simulink model "EffectuatorIntegratedWithDemonstrator"  (R2020a)
settings: Solver=FixedStepDiscrete  StartTime=0.0  StopTime=inf  FixedStep=Ts  RelTol=1e-3
InitFcn:
  | %% Verwende vordefinierte Setpoints (Kreis mit Z-Komponente)
  | 
  | % Config
  | numCircles = 3;
  | scale=6;
  | %Versuch symmetrische Setpunkte zu setzen
  | pointsPerCircle =scale*(4+3*numCircles)+2;
  | 
  | r = 50;
  | m_x = r;
  | m_y = r;
  | 
  | % //
  | s = linspace(0,2*pi,pointsPerCircle);
  | 
  | setPoints_x = [];
  | setPoints_y = [];
  | 
  | for ii=1:numCircles
  | 
  | setPoints_x = [setPoints_x (-cos(s(1:floor(pointsPerCircle / 2))).*r + m_x + 2*r*(ii-1))]; %#ok<AGROW>
  | setPoints_y = [setPoints_y (sin(s).*r+m_y)]; %#ok<AGROW>pointsPerCircle / 2
  | 
  | end
  | 
  | setPoints_x = [setPoints_x flip(setPoints_x(1:end))];
  | 
  | % Loeschen doppelter y-Werte (Kreisuebergang)
  | setPoints_x(pointsPerCircle .* [1:numCircles]) = [];
  | setPoints_y(pointsPerCircle .* [1:numCircles]) = [];
  | 
  | % setPoints_x= [linspace(0,setPoints_x(19),19) setPoints_x(20:end)];
  | % setPoints_y= [linspace(0,setPoints_y(19),19) setPoints_y(20:end)];
  | 
  | % Array Elemente verschieben
  | % setPoints_x = circshift(setPoints_x,-pointsPerCircle/4,2);
  | % setPoints_y = circshift(setPoints_y,-pointsPerCircle/4,2);
  | 
  | z = zeros(1,size(setPoints_x,2));
  | z_x = -5:5;
  | z_y = -z_x.^2 + 25;
  | z_idx = 90;
  | z_idx2 = 210;
  | z(z_idx:z_idx+length(z_x)-1) = z_y;
  | z(z_idx2:z_idx2+length(z_x)-1) = z_y;
  | % z = [z_y z];
  | setPoints_z = z;
  | 
  | % setPoints_x = [zeros(1,length(z_y)) setPoints_x];
  | % setPoints_y = [setPoints_y(1,1)*ones(1,length(z_y)) setPoints_y];
  | 
  | % Umrechnung der Einheiten für Demonstrator
  | % setPoints_x = setPoints_x ./ 1000;
  | % setPoints_y = setPoints_y ./ 1000;
  | % setPoints_z = setPoints_z ./ 1000;
  | 
  | 
  | %{
  | plot(setPoints_x,setPoints_y);
  | fig = figure;
  | plot3(setPoints_x(1:end-1),setPoints_y(1:end-1),setPoints_z(1:end-1));
  | 
  | ax = gca;
  | ax.YDir = 'reverse';
  | ax.ZDir = 'reverse';
  | %}
  | 
  | % setPoints_z = zeros(1,size(setPoints_x,2));
  | 
  | setP_mat = [setPoints_x;setPoints_y;setPoints_z];
  | %Dauerlauftest zehn Durchgänge
  | %setP_mat = repmat(setP_mat, 1, 10);
  | setP_mat = setP_mat(:,2:end);
StartFcn:
  | close all;
model workspace (MAT data in the model file):
  MvmtPerfEval_collectVal = Simulink.Parameter
  MvmtPerfEval_collectVal.Value = 0.65
  MvmtPerfEval_collectVal.Description = '- Anteil eines Interpolationssegments (0,1)
    | - Nach Abarbeitung des spezifizierten Anteils wird gemeinsame Performance aller Agenten
    | vom Dispatcher geladen
    | 
    | - (!!!) Wert MUSS größer sein als MvmtPerfEval_sendOwnVal'
  MvmtPerfEval_collectVal.DataType = 'auto'
  MvmtPerfEval_collectVal.Min = 0
  MvmtPerfEval_collectVal.Max = 1
  MvmtPerfEval_collectVal.Dimensions = [1 1]
  MvmtPerfEval_sendOwnVal = Simulink.Parameter
  MvmtPerfEval_sendOwnVal.Value = 0.6
  MvmtPerfEval_sendOwnVal.Description = '- Anteil eines Interpolationssegments (0,1)
    | - Nach Abarbeitung des spezifizierten Anteils wird Perfomance Kennzahl an Dispatcher übermittelt
    | 
    | - (!!!) Wert MUSS kleiner sein als MvmtPerfEval_collectVal'
  MvmtPerfEval_sendOwnVal.DataType = 'auto'
  MvmtPerfEval_sendOwnVal.Min = 0
  MvmtPerfEval_sendOwnVal.Max = 1
  MvmtPerfEval_sendOwnVal.Dimensions = [1 1]
  PerfEval_numTicks_enable = Simulink.Parameter
  PerfEval_numTicks_enable.Value = 10
  PerfEval_numTicks_enable.Description = 'Anzahl der Ticks (Integrationsschritte), bevor die Performance ausgewertet wird
    | (unabhängig vom Senden des Werts an den Dispatcher)'
  PerfEval_numTicks_enable.DataType = 'auto'
  PerfEval_numTicks_enable.Dimensions = [1 1]
  Segmentregler_I_Gain = Simulink.Parameter
  Segmentregler_I_Gain.Value = 1
  Segmentregler_I_Gain.DataType = 'auto'
  Segmentregler_I_Gain.Dimensions = [1 1]
  Segmentregler_P_Gain = Simulink.Parameter
  Segmentregler_P_Gain.Value = 0
  Segmentregler_P_Gain.DataType = 'auto'
  Segmentregler_P_Gain.Dimensions = [1 1]
  Segmentregler_minVel_enable = Simulink.Parameter
  Segmentregler_minVel_enable.Value = 0.1
  Segmentregler_minVel_enable.DataType = 'auto'
  Segmentregler_minVel_enable.Dimensions = [1 1]
  Segmentregler_numTicks_enable = Simulink.Parameter
  Segmentregler_numTicks_enable.Value = 30
  Segmentregler_numTicks_enable.Description = 'Anzahl der Ticks (Integrationsschritte), bevor der Segmentregler aktiv wird'
  Segmentregler_numTicks_enable.DataType = 'auto'
  Segmentregler_numTicks_enable.Dimensions = [1 1]
  Ts = Simulink.Parameter
  Ts.Value = 0.005
  Ts.Description = 'Sampling Time'
  Ts.DataType = 'auto'
  Ts.Dimensions = [1 1]
  maxPos_x = Simulink.Parameter
  maxPos_x.Value = 300
  maxPos_x.Description = 'Grenze des Arbeitsbereichs (maximaler Wert der Koordinate)'
  maxPos_x.DataType = 'auto'
  maxPos_x.Dimensions = [1 1]
  maxPos_y = Simulink.Parameter
  maxPos_y.Value = 150
  maxPos_y.Description = 'Grenze des Arbeitsbereichs (maximaler Wert der Koordinate)'
  maxPos_y.DataType = 'auto'
  maxPos_y.Dimensions = [1 1]
  maxPos_z = Simulink.Parameter
  maxPos_z.Value = 50
  maxPos_z.Description = 'Grenze des Arbeitsbereichs (maximaler Wert der Koordinate)'
  maxPos_z.DataType = 'auto'
  maxPos_z.Dimensions = [1 1]
  maxVectorLengths = Simulink.Parameter
  maxVectorLengths.Value = 16376
  maxVectorLengths.DataType = 'auto'
  maxVectorLengths.Dimensions = [1 1]
  minAllowedVelSaturation = Simulink.Parameter
  minAllowedVelSaturation.Value = 0.05
  minAllowedVelSaturation.Description = 'Minimaler Saturation-Wert für den Geschwindigkeits-PID-Regler
    | (auch bei Sollgeschwindigkeit soll Fehlerkorrektur möglich sein)'
  minAllowedVelSaturation.DataType = 'auto'
  minAllowedVelSaturation.Dimensions = [1 1]
  numAxes = Simulink.Parameter
  numAxes.Value = 4
  numAxes.DataType = 'auto'
  numAxes.Dimensions = [1 1]
undefined symbols (not defined in the file or in its folder): DiscIntNeverNeededParam, VelOverride
libraries: simulink x20, vrlib x5, sldrtlib x2, xpcrtudplib x2, dspnetwork x2, ptplib x1, etargetslib x1, xpcutilitieslib x1
(part 1 of 5)
settings Model: xpc_rtwmakecfg_data=_xpcnblib__xpcetherlib__xpcether8255xlib__xpcetherGbElib__xpciplib_  EnablePacing=on  PacingRate=10  Creator=Daniel  LastModifiedBy=Hiwi
settings DataIOCC: ReturnWorkspaceOutputs=off
settings DebuggingCC: AlgebraicLoopMsg=none  ArithmeticOperatorsInVariantConditions=warning
settings SFSimCC: CustomCodeUndefinedFunction=UseInterfaceOnly

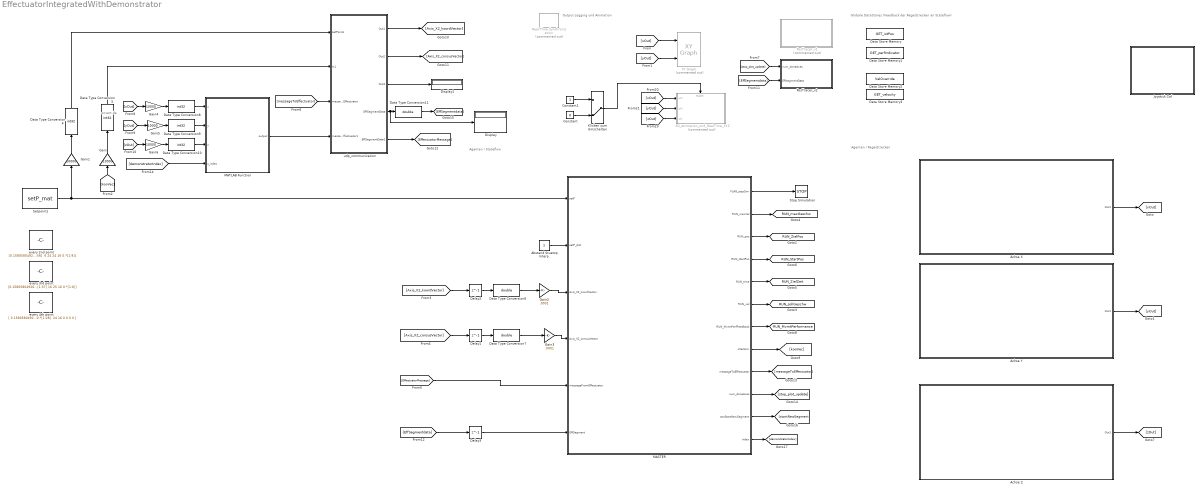
== system EffectuatorIntegratedWithDemonstrator ==
  note: onvert da
  note: Globale DataStores (Feedback der Regelstrecken an Stateflow)
  note: Agenten / Regelstrecken
  note: Agenten / Stateflow
  note: Output-Logging und Animation
  3D_Animation_und_RealTime_XYZ : Subsystem  Commented=on
  Abstand Stuetzp. Interp. : Constant
  Achse X : Subsystem
  Achse Y : Subsystem
  Achse Z : Subsystem
  Constant : Constant  Value=0
  Constant1 : Constant
  Data Store Memory : DataStoreMemory  DataStoreName=GET_istPos  ReadBeforeWriteMsg=warning  WriteAfterWriteMsg=warning  WriteAfterReadMsg=warning  InitialValue=zeros(1,numAxes)  ShowAdditionalParam=off  OutDataTypeStr=double
  Data Store Memory1 : DataStoreMemory  DataStoreName=GET_perfIndicator  ReadBeforeWriteMsg=warning  WriteAfterWriteMsg=warning  WriteAfterReadMsg=warning  InitialValue=zeros(1,numAxes)  ShowAdditionalParam=off  OutDataTypeStr=double
  Data Store Memory2 : DataStoreMemory  DataStoreName=VelOverride  ReadBeforeWriteMsg=warning  WriteAfterWriteMsg=warning  WriteAfterReadMsg=warning  InitialValue=ones(1,numAxes)  ShowAdditionalParam=off  OutDataTypeStr=double
  Data Store Memory3 : DataStoreMemory  DataStoreName=GET_velocity  ReadBeforeWriteMsg=warning  WriteAfterWriteMsg=warning  WriteAfterReadMsg=warning  InitialValue=zeros(1,numAxes)  ShowAdditionalParam=off  OutDataTypeStr=double
  Data Type Conversion{4..5,8..10} (5 alike) : DataTypeConversion  OutDataTypeStr=int32
  Data Type Conversion11 : DataTypeConversion  OutDataTypeStr=double
  Data Type Conversion6 : DataTypeConversion  OutDataTypeStr=double
  Data Type Conversion7 : DataTypeConversion  OutDataTypeStr=double
  Delay1 : Delay  DelayLength=1
  Delay2 : Delay  DelayLength=1
  Delay3 : Delay  DelayLength=1
  Display : Display
  Display1 : Display
  Gain{,1,4..6} (5 alike) : Gain  Gain=10000
  Gain2 : Gain  Gain=.0001
  Gain3 : Gain  Gain=.0001
  Joystick Ctrl : Subsystem
  Klicken zum Umschalten : ManualSwitch  CurrentSetting=0
  MASTER : Stateflow chart  TreatAsAtomicUnit=on
  MATLAB Function : MATLAB Function  TreatAsAtomicUnit=on
  PosTracer_v1 : Stateflow chart  Commented=on  TreatAsAtomicUnit=on
  PosTracer_v2 : Stateflow chart  TreatAsAtomicUnit=on
  Real-Time Synchronization : sldrtlib/Real-Time Synchronization  Commented=on  SampleTime=0.005  MaxMissedTicks=1000  ShowMissedTicks=off  YieldWhenWaiting=off
  Setpoints : Constant  Value=setP_mat
  Stop Simulation : Stop
  XY Graph : simulink/Sinks/XY Graph  Commented=on  xmin=0  xmax=maxPos_x  ymin=0  ymax=maxPos_y  st=-1
  every 2nd point : Constant  Value="[0.158058049265208 1.41653299797949 3.90170726358966 7.55083189543181 12.2717689920885 17.9453181203890 24.4282260448289 31.5568037737996 39.1510595946841 47.0192437415090 54.9626899454031 62.7808316220237 70.2762660406497 77.2597386081334 83.5549214179519 89.0028654092606 93.4660137219791 96.8316749134364 99.0148683402318 99.9604698613651 100.158058049265 101.416532997979 103.901707263590 107.550831895432 112.271768992089 117.945318120389 124.428226044829  131.556803773800 139.151059594684 147.019243741509 154.962689945403 162.780831622024 170.276266040650 177.259738608133 183.554921417952 189.002865409261 193.466013721979 196.831674913436 199.014868340232 200 200.631232903183 202.508993413611  205.585869362543 209.784171736462 214.997896271529 221.095399988758 227.922725089204 235.307486283104 243.063223400547  250.994109383254 258.899894783877 266.580963927603 273.843375071425  280.503757300526 286.393940518475 291.365201627153 295.292019683276 298.075245216371 299.644603685099 299.960469861365  299.014868340232 296.831674913436  293.466013721979 289.002865409261 283.554921417952 277.259738608133 270.276266040650 262.780831622024 254.962689945403 247.019243741509 239.151059594684 231.556803773800 224.428226044829 217.945318120389 212.271768992088 207.550831895432 203.901707263590 201.416532997980 200.158058049265 199.644603685099 198.075245216371 195.292019683276 191.365201627153 186.393940518475 180.503757300526 173.843375071425 166.580963927603 158.899894783878 150.994109383254 143.063223400547 135.307486283104 127.922725089204 121.095399988758 114.997896271529 109.784171736462 105.585869362543 102.508993413611 100.631232903183 100 99.6446036850987 98.0752452163710 95.2920196832762 91.3652016271529 86.3939405184747 80.5037573005262 73.8433750714253 66.5809639276034 58.8998947838775 50.9941093832535 43.0632234005466 35.3074862831040 27.9227250892044 21.0953999887576 14.9978962715287 9.78417173646176 5.58586936254341 2.50899341361087 0.631232903183332 ; 53.9725083485857 61.8172219266452 69.3635587325321 76.4209789226310 82.8112874635188 88.3731334346954 92.9660840289831 96.4741703848694 98.8088157209525 99.9110718390967 99.7531075261214  98.3389112729019 95.7041905677017 91.9154703065138 87.0684130849309 81.2854037830280 74.7124594308362 67.5155423781912 59.8763698588976 51.9878257548463 44.0490904099048 36.2606114624487 28.8190426795736 21.9122785839615 15.7147102456794 10.3828220269213  6.05124045887832 2.82933501389326 0.798456601078975 0.00988351149672440 0.483526676374908 2.20742692971196 5.13805696903938 9.20142039004195 14.2949200451625 20.2899485514145 27.0351355388511 34.3601696488886 42.0800987796393 50 57.9199012203608 65.6398303511114 72.9648644611489 79.7100514485855 85.7050799548375 90.7985796099580 94.8619430309606 97.7925730702880 99.5164733236251 99.9901164885033 99.2015433989211 97.1706649861067 93.9487595411217 89.6171779730787 84.2852897543207 78.0877214160385 71.1809573204264 63.7393885375513 55.9509095900952 48.0121742451537 40.1236301411024 32.4844576218088 25.2875405691639 18.7145962169720 12.9315869150691 8.08452969348616 4.29580943229828 1.66108872709815 0.246892473878624 0.0889281609033432 1.19118427904746 3.52582961513065 7.03391597101695 11.6268665653046 17.1887125364812 23.5790210773690 30.6364412674680 38.1827780733548 46.0274916514143 53.9725083485857 61.8172219266452 69.3635587325321 76.4209789226310 82.8112874635188 88.3731334346954 92.9660840289831 96.4741703848694 98.8088157209525 99.9110718390967 99.7531075261214 98.3389112729019 95.7041905677017  91.9154703065138 87.0684130849309 81.2854037830280 74.7124594308362 67.5155423781912 59.8763698588976 51.9878257548463 44.0490904099048 36.2606114624487 28.8190426795736 21.9122785839615 15.7147102456794 10.3828220269213 6.05124045887832 2.82933501389326 0.798456601078975 0.00988351149672440 0.483526676374908 2.20742692971196 5.13805696903938 9.20142039004195 14.2949200451625 20.2899485514145 27.0351355388511 34.3601696488886 42.0800987796393 ; 0.*[1:45] 16 24 24 16 0.*[1:56]  6 24 24 16 0.*[1:9]]"  VectorParams1D=off
  every 3rd point : Constant  Value="[0.158058049265208 2.50899341361087 7.55083189543181  14.9978962715287 24.4282260448289 35.3074862831040 47.0192437415090 58.8998947838775 70.2762660406497 80.5037573005262 89.0028654092606 95.2920196832762 99.0148683402318 100 101.416532997979 105.585869362543 112.271768992089 121.095399988758 131.556803773800 143.063223400547 154.962689945403 166.580963927603 177.259738608133 186.393940518475 193.466013721979 198.075245216371 200 201.416532997980 205.585869362543 212.271768992088 221.095399988758 231.556803773800 243.063223400547 254.962689945403 266.580963927603 277.259738608133 286.393940518475 293.466013721979 298.075245216371 299.960469861365 299.014868340232 295.292019683276 289.002865409261 280.503757300526 270.276266040650 258.899894783877 247.019243741509 235.307486283104 224.428226044829 214.997896271529 207.550831895432 202.508993413611 200.158058049265 199.014868340232 195.292019683276 189.002865409261 180.503757300526 170.276266040650 158.899894783878 147.019243741509 135.307486283104 124.428226044829 114.997896271529 107.550831895432 102.508993413611 100.158058049265 99.6446036850987 96.8316749134364 91.3652016271529 83.5549214179519 73.8433750714253 62.7808316220237 50.9941093832535 39.1510595946841 27.9227250892044 17.9453181203890 9.78417173646176 3.90170726358966 0.631232903183332; 53.9725083485857 65.6398303511114 76.4209789226310 85.7050799548375 92.9660840289831 97.7925730702880 99.9110718390967 99.2015433989211 95.7041905677017 89.6171779730787 81.2854037830280 71.1809573204264 59.8763698588976 48.0121742451537 36.2606114624487 25.2875405691639 15.7147102456794 8.08452969348616 2.82933501389326 0.246892473878624 0.483526676374908 3.52582961513065 9.20142039004195 17.1887125364812 27.0351355388511 38.1827780733548 50 61.8172219266452 72.9648644611489 82.81128746351 88 90.7985796099580 96.4741703848694 99.5164733236251 99.7531075261214 97.1706649861067 91.9154703065138 84.2852897543207 74.7124594308362 63.7393885375513 51.9878257548463 40.1236301411024 28.8190426795736 18.7145962169720 10.3828220269213 4.29580943229828 0.798456601078975 0.0889281609033432 2.20742692971196 7.03391597101695 14.2949200451625 23.5790210773690 34.3601696488886 46.0274916514143 57.9199012203608 69.3635587325321 79.7100514485855 88.3731334346954 94.8619430309606 98.8088157209525 99.9901164885033 98.3389112729019 93.9487595411217 87.0684130849309 78.0877214160385 67.5155423781912 55.9509095900952 44.0490904099048 32.4844576218088  21.9122785839615 12.9315869150691 6.05124045887832 1.66108872709815 0.00988351149672440 1.19118427904746 5.13805696903938 11.6268665653046 30.6364412674680 42.0800987796393;0.*[1:30] 16 25 16 0.*[1:37] 16 25 16 0.*[1:6]]"  VectorParams1D=off
  every 4th point : Constant  Value="[ 0.158058049265208 3.90170726358966 12.2717689920885 24.4282260448289 39.1510595946841 54.9626899454031 70.2762660406497 83.5549214179519  93.4660137219791 99.0148683402318 100.158058049265  103.901707263590 112.271768992089 124.428226044829 139.151059594684 154.962689945403  170.276266040650 183.554921417952 193.466013721979 199.014868340232 200.631232903183  205.585869362543 214.997896271529 227.922725089204 243.063223400547 258.899894783877 273.843375071425 286.393940518475 295.292019683276 299.644603685099 299.014868340232 293.466013721979 283.554921417952 270.276266040650 254.962689945403 239.151059594684 224.428226044829 212.271768992088 203.901707263590 200.158058049265 198.075245216371 191.365201627153 180.503757300526 166.580963927603 150.994109383254 135.307486283104 121.095399988758 109.784171736462 102.508993413611 100 98.0752452163710 91.3652016271529 80.5037573005262 66.5809639276034 50.9941093832535 35.3074862831040 21.0953999887576 9.78417173646176 2.50899341361087; 53.9725083485857 69.3635587325321 82.8112874635188 92.9660840289831 98.8088157209525 99.7531075261214 95.7041905677017 87.0684130849309 74.7124594308362 59.8763698588976 44.0490904099048 28.8190426795736 15.7147102456794 6.05124045887832 0.798456601078975 0.483526676374908 5.13805696903938 14.2949200451625 27.0351355388511  42.0800987796393 57.9199012203608 72.9648644611489  85.7050799548375 94.8619430309606 99.5164733236251 99.2015433989211  93.9487595411217 84.2852897543207 71.1809573204264 55.9509095900952 40.1236301411024 25.2875405691639 12.9315869150691  4.29580943229828 0.246892473878624  1.19118427904746 7.03391597101695 17.1887125364812 30.6364412674680 46.0274916514143 61.8172219266452 76.4209789226310 88.3731334346954 96.4741703848694 99.9110718390967 98.3389112729019 91.9154703065138  81.2854037830280 67.5155423781912 51.9878257548463 36.2606114624487 21.9122785839615 10.3828220269213 2.82933501389326 0.00988351149672440 2.20742692971196 9.20142039004195 20.2899485514145 34.3601696488886;0.*[1:23] 24 16 0.*[1:28]  24 16 0 0 0 0 ]"  VectorParams1D=off
  udp_communication : Subsystem
  tag scope: RUN_MvmtPerformance=global, RUN_StartPos=global, RUN_ZielPos=global, RUN_ZielZeit=global, RUN_maxGeschw=global, RUN_sollGeschw=global
  wires:
  Achse X/1(Out1) -> [xOut]
  [xOut] -> XY Graph/1
  [yOut] -> XY Graph/2
  Constant/1 -> Klicken zum Umschalten/2
  Constant1/1 -> Klicken zum Umschalten/1
  [xOut] -> 3D_Animation_und_RealTime_XYZ/1(xIn)
  [yOut] -> 3D_Animation_und_RealTime_XYZ/2(yIn)
  [zOut] -> 3D_Animation_und_RealTime_XYZ/3(zIn)
  MASTER/1(FLAG_stopSim) -> Stop Simulation/1
  MASTER/2(RUN_maxVel) -> [RUN_maxGeschw]
  MASTER/3(RUN_pos) -> [RUN_ZielPos]
  MASTER/4(RUN_startPos) -> [RUN_StartPos]
  MASTER/5(RUN_time) -> [RUN_ZielZeit]
  MASTER/6(RUN_vel) -> [RUN_sollGeschw]
  Achse Y/1(Out1) -> [yOut]
  Achse Z/1(Out1) -> [zOut]
  Klicken zum Umschalten/1 -> 3D_Animation_und_RealTime_XYZ/Enable
  MASTER/7(RUN_MvmtPerfFeedback) -> [RUN_MvmtPerformance]
  Data Type Conversion4/1 -> udp_communication/1(setPoints)
  [kooVec] -> Gain/1
  [Axis_X2_koordVector] -> Delay2/1
  udp_communication/1(Out1) -> [Axis_X2_koordVector]
  MASTER/8(cVectors) -> [kooVec]
  udp_communication/2(Out2) -> [Axis_X2_consusVector]
  Data Type Conversion5/1 -> udp_communication/2(In1)
  [Axis_X2_consusVector] -> Delay1/1
  Delay1/1 -> Data Type Conversion7/1
  Data Type Conversion6/1 -> Gain2/1
  Data Type Conversion7/1 -> Gain3/1
  Gain/1 -> Data Type Conversion5/1
  Gain1/1 -> Data Type Conversion4/1
  Gain2/1 -> MASTER/3(Axis_X2_koordVector)
  Gain3/1 -> MASTER/4(Axis_X2_consusVector)
  [EffectuatorMessage] -> MASTER/5(messageFromEffectuator)
  MASTER/9(messageToEffectuator) -> [messageToEffectuator]
  Abstand Stuetzp. Interp./1 -> MASTER/2(setP_dist)
  Delay2/1 -> Data Type Conversion6/1
  [messageToEffectuator] -> udp_communication/3(messageToEffectuator)
  Setpoints/1 -> Gain1/1, MASTER/1(setP)
  udp_communication/3(Out3) -> Display1/1
  MASTER/10(num_doneAxes) -> [stop_plot_update]
  [stop_plot_update] -> PosTracer_v2/1(num_doneAxes)
  [xOut] -> Gain4/1
  [yOut] -> Gain5/1
  [zOut] -> Gain6/1
  Gain4/1 -> Data Type Conversion8/1
  Gain5/1 -> Data Type Conversion9/1
  Gain6/1 -> Data Type Conversion10/1
  Data Type Conversion8/1 -> MATLAB Function/1(x)
  Data Type Conversion9/1 -> MATLAB Function/2(y)
  Data Type Conversion10/1 -> MATLAB Function/3(z)
  MATLAB Function/1(output) -> udp_communication/4(messageToEffectuator1)
  udp_communication/5(EffSegmentData1) -> [EffectuatorMessage]
  udp_communication/4(EffSegmentData) -> Display/1, Data Type Conversion11/1
  Data Type Conversion11/1 -> [EffSegmentdata]
  [EffSegmentdata] -> PosTracer_v2/2(EffsegmentData)
  [EffSegmentdata] -> Delay3/1
  Delay3/1 -> MASTER/6(EffSegment)
  MASTER/11(canStartNewSegment) -> [startNewSegment]
  MASTER/12(index) -> [demonstratorIndex]
  [demonstratorIndex] -> MATLAB Function/4(s_index)

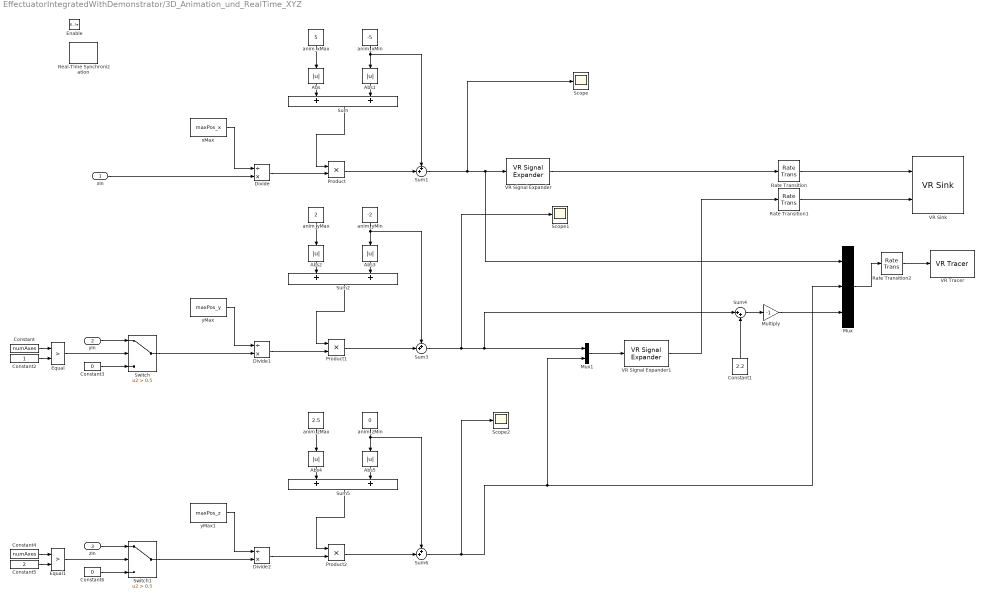
== system EffectuatorIntegratedWithDemonstrator/3D_Animation_und_RealTime_XYZ ==
  xIn : Inport
  yIn : Inport  Port=2
  zIn : Inport  Port=3
  Enable : EnablePort
  Abs{,1..5} (6 alike) : Abs
  Constant : Constant  Value=numAxes
  Constant1 : Constant  Value=2.2
  Constant2 : Constant
  Constant3 : Constant  Value=0
  Constant4 : Constant  Value=numAxes
  Constant5 : Constant  Value=2
  Constant6 : Constant  Value=0
  Divide : Product  Inputs=/*
  Divide1 : Product  Inputs=/*
  Divide2 : Product  Inputs=/*
  Equal : RelationalOperator  Operator=>  OutDataTypeStr=boolean  RndMeth=Simplest
  Equal1 : RelationalOperator  Operator=>  OutDataTypeStr=boolean  RndMeth=Simplest
  Multiply : Gain  Gain=-1
  Mux : Mux  Inputs=3
  Mux1 : Mux  Inputs=2
  Product : Product
  Product1 : Product
  Product2 : Product
  Rate Transition : RateTransition  OutPortSampleTime=0.1
  Rate Transition1 : RateTransition  OutPortSampleTime=0.1
  Rate Transition2 : RateTransition  OutPortSampleTime=0.3
  Real-Time Synchronization : sldrtlib/Real-Time Synchronization  SampleTime=0.005  MaxMissedTicks=1000  ShowMissedTicks=off  YieldWhenWaiting=off
  Scope : Scope
  Scope1 : Scope
  Scope2 : Scope
  Sum : Sum
  Sum1 : Sum  Inputs=++|
  Sum2 : Sum
  Sum3 : Sum  Inputs=++|
  Sum4 : Sum  Inputs=|++
  Sum5 : Sum
  Sum6 : Sum  Inputs=++|
  Switch : Switch  Criteria=u2 > Threshold  Threshold=0.5
  Switch1 : Switch  Criteria=u2 > Threshold  Threshold=0.5
  VR Signal Expander : vrlib/VR Signal Expander  outwidth=3  outidx=1
  VR Signal Expander1 : vrlib/VR Signal Expander  outwidth=3  outidx=[1 2]
  VR Sink : vrlib/VR Sink  InstantiateOnLoad=on  SampleTime=-1  ViewEnable=on  RemoteChange=off  RemoteView=off  FieldsWritten=yAchse.translation.3.1.1.double#TCP.translation.3.1.1.double  WorldFileName=DS_MA_3dworld.wrl  WorldDescription=DS_MA_3dworld  AutoView=on  VideoDimensions=[]  AllowVariableSize=off  FigureProperties="{'Position', 'Name', 'Viewpoint', 'CameraBound', 'CameraDirection', 'CameraPosition', 'CameraUpVector', 'ZoomFactor', 'Antialiasing', 'Headlight', 'Lighting', 'NavPanel', 'Sound', 'StatusBar', 'Stereo3D', 'Stereo3DCameraOffset', 'Stereo3DHIT', 'ToolBar', 'Textures', 'Transparency', 'Triad', 'Wireframe', 'NavZones', 'NavMode', 'NavSpeed', 'CaptureFileFormat', 'CaptureFileName', 'Record2DCompressMethod', 'Record2DCompressQuality', 'Record2D', 'Record2DFileName', 'Record2DFPS'; [2.0000000000000000e+00   9.2000000000000000e+01   5.7600000000000000e+02   3.5000000000000000e+02], 'DS_MA_3dworld', '_untitled_1', 'on', [0.0000000000000000e+00   0.0000000000000000e+00  -1.0000000000000000e+00], [0.0000000000000000e+00   0.0000000000000000e+00   0.0000000000000000e+00], [0.0000000000000000e+00   1.0000000000000000e+00   0.0000000000000000e+00], [1.0000000000000000e+00], 'on', 'on', 'on', 'halfbar', 'on', 'on', 'off', [1.0000000149011612e-01], [0.0000000000000000e+00], 'on', 'on', 'on', 'none', 'off', 'off', 'fly', 'normal', 'tif', '%f_anim_%n.tif', 'auto', [7.5000000000000000e+01], 'off', '%f_anim_%n.avi', 'auto'}"
  VR Tracer : vrlib/VR Tracer  VrmlFile=DS_MA_3dworld.wrl  MarkerName=Tetrahedron  UseLines=on  UseTriads=on  MarkerScale=[0.1 0.1 0.1]  MarkerColorSelection=Selected from color list  MarkerColor=red  rgbval=[1 0 0]  Ts=0.3  ForceViewerOpen=off  ConnectPlane=off  PlaneCoeff=[0 1 0 0]  ConnectPoint=None  PointCoord=[0 0 0]
      settings: SourceProductBaseCode=SL
  anim_xMax : Constant  Value=5
  anim_xMin : Constant  Value=-5
  anim_yMax : Constant  Value=2
  anim_yMin : Constant  Value=-2
  anim_zMax : Constant  Value=2.5
  anim_zMin : Constant  Value=0
  xMax : Constant  Value=maxPos_x
  yMax : Constant  Value=maxPos_y
  yMax1 : Constant  Value=maxPos_z
  wires:
  Constant1/1 -> Sum4/2
  Sum4/1 -> Multiply/1
  Multiply/1 -> Mux/3
  Rate Transition2/1 -> VR Tracer/1
  Mux/1 -> Rate Transition2/1
  Rate Transition1/1 -> VR Sink/2
  Rate Transition/1 -> VR Sink/1
  VR Signal Expander/1 -> Rate Transition/1
  VR Signal Expander1/1 -> Rate Transition1/1
  Sum3/1 -> Mux1/1, Sum4/1, Scope1/1
  Sum1/1 -> VR Signal Expander/1, Mux/1, Scope/1
  Switch/1 -> Divide1/2
  yMax/1 -> Divide1/1
  anim_yMax/1 -> Abs2/1
  anim_yMin/1 -> Sum3/1, Abs3/1
  Abs2/1 -> Sum2/1
  Abs3/1 -> Sum2/2
  Divide1/1 -> Product1/2
  Sum2/1 -> Product1/1
  Product1/1 -> Sum3/2
  Product/1 -> Sum1/2
  Sum/1 -> Product/1
  Divide/1 -> Product/2
  Abs1/1 -> Sum/2
  Abs/1 -> Sum/1
  anim_xMin/1 -> Abs1/1, Sum1/1
  anim_xMax/1 -> Abs/1
  xMax/1 -> Divide/1
  xIn/1 -> Divide/2
  Product2/1 -> Sum6/2
  Sum5/1 -> Product2/1
  Divide2/1 -> Product2/2
  Abs5/1 -> Sum5/2
  Abs4/1 -> Sum5/1
  anim_zMin/1 -> Abs5/1, Sum6/1
  anim_zMax/1 -> Abs4/1
  yMax1/1 -> Divide2/1
  Switch1/1 -> Divide2/2
  Sum6/1 -> Scope2/1, Mux1/2, Mux/2
  Mux1/1 -> VR Signal Expander1/1
  Constant/1 -> Equal/1
  Constant2/1 -> Equal/2
  yIn/1 -> Switch/1
  Equal/1 -> Switch/2
  Constant3/1 -> Switch/3
  Constant6/1 -> Switch1/3
  Equal1/1 -> Switch1/2
  zIn/1 -> Switch1/1
  Constant5/1 -> Equal1/2
  Constant4/1 -> Equal1/1

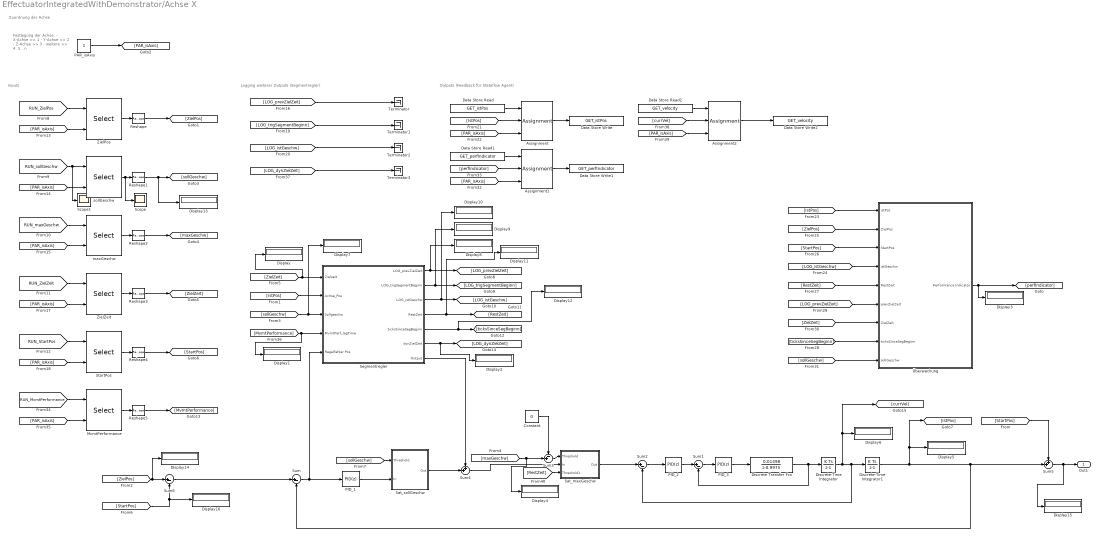
== system EffectuatorIntegratedWithDemonstrator/Achse X ==
  note: Outputs (Feedback für Stateflow Agent)
  note: Logging weiterer Outputs (Segmentregler)
  note: Zuordnung der Achse
  note: Festlegung der Achse:
      | - X-Achse >> 1
      | - Y-Achse >> 2
      | - Z-Achse >> 3
      | - weitere >> 4..5...n
  note: Inputs
  Assignment : Assignment  DiagnosticForDimensions=Warning  IndexOptions=Index vector (port)  Indices=1  OutputSizes=1
  Assignment1 : Assignment  DiagnosticForDimensions=Warning  IndexOptions=Index vector (port)  Indices=1  OutputSizes=1
  Assignment2 : Assignment  DiagnosticForDimensions=Warning  IndexOptions=Index vector (port)  Indices=1  OutputSizes=1
  Constant : Constant  Value=0
  Data Store Read : DataStoreRead  DataStoreName=GET_istPos
  Data Store Read1 : DataStoreRead  DataStoreName=GET_perfIndicator
  Data Store Read2 : DataStoreRead  DataStoreName=GET_velocity
  Data Store Write : DataStoreWrite  DataStoreName=GET_istPos
  Data Store Write1 : DataStoreWrite  DataStoreName=GET_perfIndicator
  Data Store Write2 : DataStoreWrite  DataStoreName=GET_velocity
  Discrete Transfer Fcn : DiscreteTransferFcn  Numerator=0.01498  Denominator=[1 -0.9975]
  Discrete-Time Integrator : DiscreteIntegrator  SampleTime=-1  ICPrevOutput=DiscIntNeverNeededParam  ICPrevScaledInput=DiscIntNeverNeededParam
  Discrete-Time Integrator1 : DiscreteIntegrator  SampleTime=-1  ICPrevOutput=DiscIntNeverNeededParam  ICPrevScaledInput=DiscIntNeverNeededParam
  Display{,1..16} (17 alike) : Display
  MvmtPerformance : Selector  IndexOptions=Index vector (port)  Indices=[1 3]  OutputSizes=1
  PAR_isAxis : Constant
  PID_1 : simulink/Continuous/PID Controller  Controller=PID  Form=Parallel  TimeDomain=Discrete-time  UseExternalTs=off  SampleTime=-1  IntegratorMethod=Forward Euler  FilterMethod=Forward Euler  ControllerParametersSource=internal  P=20  I=0  D=0  UseFilter=on  N=100  TunerSelectOption=Transfer Function Based (PID Tuner App)  InitialConditionSource=internal  InitialConditionForIntegrator=0  InitialConditionForFilter=0  DifferentiatorICPrevScaledInput=0  ExternalReset=none  TrackingMode=off  Kt=1  LimitOutput=off  UpperSaturationLimit=inf  LowerSaturationLimit=-inf  LinearizeAsGain=off  AntiWindupMode=none  Kb=1  POutMin=[]  POutMax=[]  IOutMin=[]  IOutMax=[]  DOutMin=[]  DOutMax=[]  NOutMin=[]  NOutMax=[]  SumOutMin=[]  SumOutMax=[]  SaturationOutMin=[]  SaturationOutMax=[]  PParamMin=[]  PParamMax=[]  IParamMin=[]  IParamMax=[]  DParamMin=[]  DParamMax=[]  NParamMin=[]  NParamMax=[]  KbParamMin=[]  KbParamMax=[]  KtParamMin=[]  KtParamMax=[]  KbOutMin=[]  KbOutMax=[]  KtOutMin=[]  KtOutMax=[]  IntegratorOutMin=[]  IntegratorOutMax=[]  FilterOutMin=[]  FilterOutMax=[]  SumI1OutMin=[]  SumI1OutMax=[]  SumI2OutMin=[]  SumI2OutMax=[]  SumI3OutMin=[]  SumI3OutMax=[]  SumI4OutMin=[]  SumI4OutMax=[]  SumDOutMin=[]  SumDOutMax=[]  DifferentiatorOutMin=[]  DifferentiatorOutMax=[]  FilterDiffOutCoefMin=[]  FilterDiffOutCoefMax=[]  ReciprocalOutMin=[]  ReciprocalOutMax=[]  SumDenOutMin=[]  SumDenOutMax=[]  SumNumOutMin=[]  SumNumOutMax=[]  DivideOutMin=[]  DivideOutMax=[]  UdiffTsProdOutMin=[]  UdiffTsProdOutMax=[]  NTsProdOutMin=[]  NTsProdOutMax=[]  UintegralTsProdOutMin=[]  UintegralTsProdOutMax=[]  UngainTsProdOutMin=[]  UngainTsProdOutMax=[]  IntegratorContinuousStateAttributes=''  IntegratorStateMustResolveToSignalObject=off  IntegratorRTWStateStorageClass=Auto  FilterContinuousStateAttributes=''  FilterStateMustResolveToSignalObject=off  FilterRTWStateStorageClass=Auto  ParallelPVariant=InternalParameters  IdealPVariant=Disabled  IVariant=InternalParameters  DVariant=InternalParameters  IntegratorVariant=Discrete  SatVariant=Disabled  AWVariant=Passthrough  PCopyVariant=Disabled  TRVariant=Disabled  FdbkBlocksVariant=Forward  IdealPFdbkVariant=Disabled  SatFdbkVariant=Disabled  DerivativeFilterVariant=ForwardEulerFilter  NVariant=InternalParameters  NCopyVariant=Disabled  FilterICVariant=InternalICsFilter  IntegratorICVariant=InternalICs  ExternalResetVariant=Disabled  TRSumVariant=Passthrough  SumFdbkVariant=Disabled  SumVariant=Sum_PID  TsampFilterVariant=InternalTs  TsampNgainVariant=Passthrough  TsampIntegralVariant=Passthrough
  PID_2 : simulink/Continuous/PID Controller  Controller=PID  Form=Parallel  TimeDomain=Discrete-time  UseExternalTs=off  SampleTime=-1  IntegratorMethod=Forward Euler  FilterMethod=Forward Euler  ControllerParametersSource=internal  P=20  I=1  D=0  UseFilter=on  N=100  TunerSelectOption=Transfer Function Based (PID Tuner App)  InitialConditionSource=internal  InitialConditionForIntegrator=0  InitialConditionForFilter=0  DifferentiatorICPrevScaledInput=0  ExternalReset=none  TrackingMode=off  Kt=1  LimitOutput=off  UpperSaturationLimit=inf  LowerSaturationLimit=-inf  LinearizeAsGain=off  AntiWindupMode=none  Kb=1  POutMin=[]  POutMax=[]  IOutMin=[]  IOutMax=[]  DOutMin=[]  DOutMax=[]  NOutMin=[]  NOutMax=[]  SumOutMin=[]  SumOutMax=[]  SaturationOutMin=[]  SaturationOutMax=[]  PParamMin=[]  PParamMax=[]  IParamMin=[]  IParamMax=[]  DParamMin=[]  DParamMax=[]  NParamMin=[]  NParamMax=[]  KbParamMin=[]  KbParamMax=[]  KtParamMin=[]  KtParamMax=[]  KbOutMin=[]  KbOutMax=[]  KtOutMin=[]  KtOutMax=[]  IntegratorOutMin=[]  IntegratorOutMax=[]  FilterOutMin=[]  FilterOutMax=[]  SumI1OutMin=[]  SumI1OutMax=[]  SumI2OutMin=[]  SumI2OutMax=[]  SumI3OutMin=[]  SumI3OutMax=[]  SumI4OutMin=[]  SumI4OutMax=[]  SumDOutMin=[]  SumDOutMax=[]  DifferentiatorOutMin=[]  DifferentiatorOutMax=[]  FilterDiffOutCoefMin=[]  FilterDiffOutCoefMax=[]  ReciprocalOutMin=[]  ReciprocalOutMax=[]  SumDenOutMin=[]  SumDenOutMax=[]  SumNumOutMin=[]  SumNumOutMax=[]  DivideOutMin=[]  DivideOutMax=[]  UdiffTsProdOutMin=[]  UdiffTsProdOutMax=[]  NTsProdOutMin=[]  NTsProdOutMax=[]  UintegralTsProdOutMin=[]  UintegralTsProdOutMax=[]  UngainTsProdOutMin=[]  UngainTsProdOutMax=[]  IntegratorContinuousStateAttributes=''  IntegratorStateMustResolveToSignalObject=off  IntegratorRTWStateStorageClass=Auto  FilterContinuousStateAttributes=''  FilterStateMustResolveToSignalObject=off  FilterRTWStateStorageClass=Auto  ParallelPVariant=InternalParameters  IdealPVariant=Disabled  IVariant=InternalParameters  DVariant=InternalParameters  IntegratorVariant=Discrete  SatVariant=Disabled  AWVariant=Passthrough  PCopyVariant=Disabled  TRVariant=Disabled  FdbkBlocksVariant=Forward  IdealPFdbkVariant=Disabled  SatFdbkVariant=Disabled  DerivativeFilterVariant=ForwardEulerFilter  NVariant=InternalParameters  NCopyVariant=Disabled  FilterICVariant=InternalICsFilter  IntegratorICVariant=InternalICs  ExternalResetVariant=Disabled  TRSumVariant=Passthrough  SumFdbkVariant=Disabled  SumVariant=Sum_PID  TsampFilterVariant=InternalTs  TsampNgainVariant=Passthrough  TsampIntegralVariant=Passthrough
  PID_3 : simulink/Continuous/PID Controller  Controller=PID  Form=Parallel  TimeDomain=Discrete-time  UseExternalTs=off  SampleTime=-1  IntegratorMethod=Forward Euler  FilterMethod=Forward Euler  ControllerParametersSource=internal  P=20  I=1  D=0  UseFilter=on  N=100  TunerSelectOption=Transfer Function Based (PID Tuner App)  InitialConditionSource=internal  InitialConditionForIntegrator=0  InitialConditionForFilter=0  DifferentiatorICPrevScaledInput=0  ExternalReset=none  TrackingMode=off  Kt=1  LimitOutput=off  UpperSaturationLimit=inf  LowerSaturationLimit=-inf  LinearizeAsGain=off  AntiWindupMode=none  Kb=1  POutMin=[]  POutMax=[]  IOutMin=[]  IOutMax=[]  DOutMin=[]  DOutMax=[]  NOutMin=[]  NOutMax=[]  SumOutMin=[]  SumOutMax=[]  SaturationOutMin=[]  SaturationOutMax=[]  PParamMin=[]  PParamMax=[]  IParamMin=[]  IParamMax=[]  DParamMin=[]  DParamMax=[]  NParamMin=[]  NParamMax=[]  KbParamMin=[]  KbParamMax=[]  KtParamMin=[]  KtParamMax=[]  KbOutMin=[]  KbOutMax=[]  KtOutMin=[]  KtOutMax=[]  IntegratorOutMin=[]  IntegratorOutMax=[]  FilterOutMin=[]  FilterOutMax=[]  SumI1OutMin=[]  SumI1OutMax=[]  SumI2OutMin=[]  SumI2OutMax=[]  SumI3OutMin=[]  SumI3OutMax=[]  SumI4OutMin=[]  SumI4OutMax=[]  SumDOutMin=[]  SumDOutMax=[]  DifferentiatorOutMin=[]  DifferentiatorOutMax=[]  FilterDiffOutCoefMin=[]  FilterDiffOutCoefMax=[]  ReciprocalOutMin=[]  ReciprocalOutMax=[]  SumDenOutMin=[]  SumDenOutMax=[]  SumNumOutMin=[]  SumNumOutMax=[]  DivideOutMin=[]  DivideOutMax=[]  UdiffTsProdOutMin=[]  UdiffTsProdOutMax=[]  NTsProdOutMin=[]  NTsProdOutMax=[]  UintegralTsProdOutMin=[]  UintegralTsProdOutMax=[]  UngainTsProdOutMin=[]  UngainTsProdOutMax=[]  IntegratorContinuousStateAttributes=''  IntegratorStateMustResolveToSignalObject=off  IntegratorRTWStateStorageClass=Auto  FilterContinuousStateAttributes=''  FilterStateMustResolveToSignalObject=off  FilterRTWStateStorageClass=Auto  ParallelPVariant=InternalParameters  IdealPVariant=Disabled  IVariant=InternalParameters  DVariant=InternalParameters  IntegratorVariant=Discrete  SatVariant=Disabled  AWVariant=Passthrough  PCopyVariant=Disabled  TRVariant=Disabled  FdbkBlocksVariant=Forward  IdealPFdbkVariant=Disabled  SatFdbkVariant=Disabled  DerivativeFilterVariant=ForwardEulerFilter  NVariant=InternalParameters  NCopyVariant=Disabled  FilterICVariant=InternalICsFilter  IntegratorICVariant=InternalICs  ExternalResetVariant=Disabled  TRSumVariant=Passthrough  SumFdbkVariant=Disabled  SumVariant=Sum_PID  TsampFilterVariant=InternalTs  TsampNgainVariant=Passthrough  TsampIntegralVariant=Passthrough
  Reshape{,1..5} (6 alike) : Reshape
  Sat_maxGeschw : Subsystem
  Sat_sollGeschw : Subsystem
  Scope : Scope
  Scope1 : Scope
  Segmentregler : Subsystem
  StartPos : Selector  IndexOptions=Index vector (port)  Indices=[1 3]  OutputSizes=1
  Sum{,1..2,6} (4 alike) : Sum  Inputs=|+-
  Sum3 : Sum  Inputs=-+|
  Sum4 : Sum  Inputs=++|
  Sum5 : Sum  Inputs=++|
  Terminator{,1..3} (4 alike) : Terminator
  ZielPos : Selector  IndexOptions=Index vector (port)  Indices=[1 3]  OutputSizes=1
  ZielZeit : Selector  IndexOptions=Index vector (port)  Indices=[1 3]  OutputSizes=1
  maxGeschw : Selector  IndexOptions=Index vector (port)  Indices=[1 3]  OutputSizes=1
  sollGeschw : Selector  IndexOptions=Index vector (port)  Indices=[1 3]  OutputSizes=1
  Überwachung : Subsystem
  Out1 : Outport  VectorParamsAs1DForOutWhenUnconnected=off
  wires:
  Sum/1 -> Segmentregler/5(Regelfehler Pos), PID_1/1
  PID_1/1 -> Sat_sollGeschw/2(In)
  Sat_sollGeschw/1(Out) -> Sum4/2
  Sum4/1 -> Sat_maxGeschw/2(In)
  PID_3/1 -> Discrete Transfer Fcn/1
  Discrete Transfer Fcn/1 -> Discrete-Time Integrator/1, Sum1/2
  Sum2/1 -> PID_2/1
  Sum6/1 -> Sum/1
  Discrete-Time Integrator/1 -> Display6/1, [currVel], Discrete-Time Integrator1/1, Sum2/2
  Sum1/1 -> PID_3/1
  PID_2/1 -> Sum1/1
  Sat_maxGeschw/1(Out) -> Sum2/1
  Discrete-Time Integrator1/1 -> Display5/1, [IstPos], Sum5/2, Sum/2
  Sum5/1 -> Display15/1, Out1/1
  [ZielPos] -> Display14/1, Sum6/1
  [ZielZeit] -> Display/1, Segmentregler/1(Zielzeit)
  [IstPos] -> Segmentregler/2(Achse_Pos)
  [StartPos] -> Sum5/1
  [StartPos] -> Display16/1, Sum6/2
  [sollGeschw] -> Display7/1, Segmentregler/3(Sollgeschw)
  [sollGeschw] -> Sat_sollGeschw/1(Threshold)
  PAR_isAxis/1 -> [PAR_isAxis]
  [PAR_isAxis] -> ZielPos/2
  [RUN_ZielPos] -> ZielPos/1
  ZielPos/1 -> Reshape/1
  sollGeschw/1 -> Scope/1, Reshape1/1
  [RUN_sollGeschw] -> Scope1/1, sollGeschw/1
  [PAR_isAxis] -> sollGeschw/2
  [PAR_isAxis] -> maxGeschw/2
  [RUN_maxGeschw] -> maxGeschw/1
  maxGeschw/1 -> Reshape2/1
  ZielZeit/1 -> Reshape3/1
  [RUN_ZielZeit] -> ZielZeit/1
  [PAR_isAxis] -> ZielZeit/2
  [PAR_isAxis] -> StartPos/2
  [RUN_StartPos] -> StartPos/1
  StartPos/1 -> Reshape4/1
  Segmentregler/1(LOG_prevZielZeit) -> Display8/1, [LOG_prevZielZeit]
  Segmentregler/2(LOG_trigSegmentBeginn) -> Display9/1, [LOG_trigSegmentBeginn]
  Segmentregler/3(LOG_istGeschw) -> Display10/1, [LOG_istGeschw]
  [LOG_prevZielZeit] -> Terminator/1
  [LOG_trigSegmentBeginn] -> Terminator1/1
  Reshape/1 -> [ZielPos]
  Reshape1/1 -> Display13/1, [sollGeschw]
  Reshape2/1 -> [maxGeschw]
  Reshape4/1 -> [StartPos]
  Reshape3/1 -> [ZielZeit]
  Data Store Read/1 -> Assignment/1
  [IstPos] -> Assignment/2
  [PAR_isAxis] -> Assignment/3
  Assignment/1 -> Data Store Write/1
  Segmentregler/4(RestZeit) -> Display11/1, [RestZeit]
  [maxGeschw] -> Display4/1, Sum3/2
  Sum3/1 -> Sat_maxGeschw/1(Threshold)
  Constant/1 -> Sum3/1
  [IstPos] -> Überwachung/1(istPos)
  [ZielPos] -> Überwachung/2(ZielPos)
  [StartPos] -> Überwachung/3(StartPos)
  [LOG_istGeschw] -> Überwachung/4(istGeschw)
  [RestZeit] -> Überwachung/5(RestZeit)
  [LOG_prevZielZeit] -> Überwachung/6(prevZielZeit)
  [ZielZeit] -> Überwachung/7(ZielZeit)
  Assignment1/1 -> Data Store Write1/1
  [PAR_isAxis] -> Assignment1/3
  [perfIndicator] -> Assignment1/2
  Data Store Read1/1 -> Assignment1/1
  Überwachung/1(Performance Indicator) -> Display3/1, [perfIndicator]
  Segmentregler/5(ticksSinceSegBeginn) -> Display12/1, [ticksSinceSegBeginn]
  [ticksSinceSegBeginn] -> Überwachung/8(ticksSinceSegBeginn)
  [sollGeschw] -> Überwachung/9(sollGeschw)
  Reshape5/1 -> [MvmtPerformance]
  MvmtPerformance/1 -> Reshape5/1
  [RUN_MvmtPerformance] -> MvmtPerformance/1
  [PAR_isAxis] -> MvmtPerformance/2
  [MvmtPerformance] -> Display1/1, Segmentregler/4(MvmtPerf_lagTime)
  Segmentregler/6(dynZielZeit) -> Display2/1, [LOG_dynZielZeit]
  [LOG_dynZielZeit] -> Terminator3/1
  [PAR_isAxis] -> Assignment2/3
  [currVel] -> Assignment2/2
  Data Store Read2/1 -> Assignment2/1
  Assignment2/1 -> Data Store Write2/1
  [LOG_istGeschw] -> Terminator2/1
  Segmentregler/7(Output) -> Sum4/1
  [RestZeit] -> Sat_maxGeschw/3(Threshold1)
